simulink model "LKAS_AutoSave_DF_20220408_1006_SW62"  (R2018b)
settings: Solver=FixedStepDiscrete  StartTime=0.0  StopTime=10.0  FixedStep=0.01  RelTol=1e-3
undefined symbols (not defined in the file): LKA_CarWidth, LKA_SampleTime, LKA_StrRatio_C, LKA_Veh2CamL_C, LKA_Veh2CamW_C, LKA_WhlBaseL_C, LL_CompHdAg_C, LL_CompSWA_C, LL_CrvtPrvwT_C, LL_DesDvt_C, LL_DvtComp_C, LL_DvtPrvwT_C, LL_DvtSpdDet_vDvtSpdMin_C, LL_HandsOff_ExitTime, LL_HandsOff_TextTime, LL_HandsOff_WarnTime, LL_HdAgExT_C, LL_HdAgPrvwT_C, LL_LAccMax_C, LL_LAccRMax_C, LL_LDW_EarliestWarnLine_C, LL_LDW_LatestWarnLine_C, LL_LDWS_SUPPRESS_HEADING, LL_LFClb_TFC_FfCtlRatio_C, LL_LFClb_TFC_KdBalance_C, LL_LFClb_TFC_KdMaxSWA_C, LL_LFClb_TFC_KdV1_C, LL_LFClb_TFC_KdV2_C, LL_LFClb_TFC_KdVehSpdLwr_C, LL_LFClb_TFC_KdVehSpdUpr_C, LL_LFClb_TFC_Ki_C, LL_LFClb_TFC_KiMaxSWA_C, LL_LFClb_TFC_Kp_C, LL_LFClb_TFC_KpKlat_C, LL_LFClb_TFC_KpV1_C, LL_LFClb_TFC_KpV2_C, LL_LFClb_TFC_KpVehSpdLwr_C, LL_LFClb_TFC_KpVehSpdUpr_C, LL_LFClb_TFC_PrvwT_C, LL_LKA_EarliestWarnLine_C, LL_LKA_LatestWarnLine_C, LL_LKAExPrcs_ExitC0Dvt, LL_LKAExPrcs_ExitC0Swt, LL_LKAExPrcs_tiExitDelayTime3, LL_LKAExPrcs_tiExitTime1, LL_LKAExPrcs_tiExitTime2, LL_LKAExPrcs_tiExitTime3, LL_LKAS_OUT_OF_CONTROL_LAT_VEL, LL_LKAS_OUT_OF_CONTROL_TTLC, LL_LKASWASyn_M0, LL_LKASWASyn_M1, LL_LKASWASyn_M2, LL_LKASWASyn_M3D, LL_LKASWASyn_M3K_DT, LL_LKASWASyn_M3K_MSD, LL_LKASWASyn_M4K, LL_LKASWASyn_SWAaddMax, LL_LKASWASyn_T2, LL_LKASWASyn_tiTrqSwaRtTime, LL_LKASWASyn_tiTrqSwaTime ... (+47)
libraries: simulink x234, canmsglib x6, dspstat3 x3, simulink_extras x1
(part 7 of 16)

== system LKAS_AutoSave_DF_20220408_1006_SW62/LKAS/LL/LL Inputs Mapping/bsLaneInfo/LanesReconstruct /Right Lane Reconstruct (RgtLaneR) ==
  bsL0Info : Inport
  bsR0Info : Inport  Port=2
  lRoadW : Inport  Port=3
  Add : Sum  OutDataTypeStr=single
  Bus Creator1 : BusCreator  Inputs=8
  Bus Selector1 : BusSelector  OutputSignals=R0_Q
  Bus Selector3 : BusSelector  OutputSignals=L0_C0,L0_C1,L0_C2,L0_C3,L0_VR,L0_Type,L0_W
  Cast To Single{1..4,6} (5 alike) : DataTypeConversion  OutDataTypeStr=single  LockScale=on
  Cast To Single5 : DataTypeConversion  OutDataTypeStr=uint8  LockScale=on
  bsR0InfoR : Outport
  wires:
  Cast To Single4/1 -> Bus Creator1/5  "R0_VR"
  Cast To Single3/1 -> Bus Creator1/4  "R0_C3"
  Cast To Single2/1 -> Bus Creator1/3  "R0_C2"
  Cast To Single1/1 -> Bus Creator1/2  "R0_C1"
  Add/1 -> Bus Creator1/1  "R0_C0"
  Bus Creator1/1 -> bsR0InfoR/1  "bsR0Info"
  Bus Selector1/1 -> Bus Creator1/6  "<R0_Q>"
  bsR0Info/1 -> Bus Selector1/1
  Bus Selector3/5 -> Cast To Single4/1  "<L0_VR>"
  Bus Selector3/4 -> Cast To Single3/1  "<L0_C3>"
  Bus Selector3/3 -> Cast To Single2/1  "<L0_C2>"
  Bus Selector3/2 -> Cast To Single1/1  "<L0_C1>"
  lRoadW/1 -> Add/1
  bsL0Info/1 -> Bus Selector3/1
  Bus Selector3/1 -> Add/2  "<L0_C0>"
  Bus Selector3/6 -> Cast To Single5/1  "<L0_Type>"
  Bus Selector3/7 -> Cast To Single6/1  "<L0_W>"
  Cast To Single5/1 -> Bus Creator1/7  "R0_Type"
  Cast To Single6/1 -> Bus Creator1/8  "R0_W"

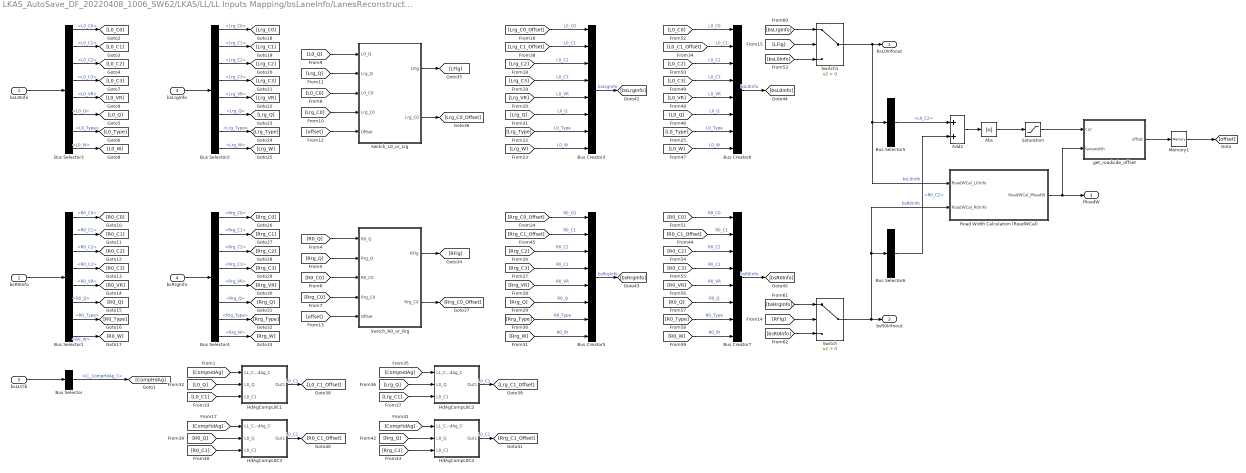
== system LKAS_AutoSave_DF_20220408_1006_SW62/LKAS/LL/LL Inputs Mapping/bsLaneInfo/LanesReconstruct /RoadSide Offset ==
  bsL0Info : Inport
  bsR0Info : Inport  Port=2
  bsLrgInfo : Inport  Port=3
  bsRrgInfo : Inport  Port=4
  bsLLClb : Inport  Port=5
  Abs : Abs
  Add2 : Sum
  Bus Creator{3,5..7} (4 alike) : BusCreator  Inputs=8
  Bus Selector : BusSelector  OutputSignals=bsLKAClb.LL_CompHdAg_C
  Bus Selector1 : BusSelector  OutputSignals=R0_C0,R0_C1,R0_C2,R0_C3,R0_VR,R0_Q,R0_Type,R0_W
  Bus Selector2 : BusSelector  OutputSignals=Lrg_C0,Lrg_C1,Lrg_C2,Lrg_C3,Lrg_VR,Lrg_Q,Lrg_Type,Lrg_W
  Bus Selector3 : BusSelector  OutputSignals=L0_C0,L0_C1,L0_C2,L0_C3,L0_VR,L0_Q,L0_Type,L0_W
  Bus Selector4 : BusSelector  OutputSignals=Rrg_C0,Rrg_C1,Rrg_C2,Rrg_C3,Rrg_VR,Rrg_Q,Rrg_Type,Rrg_W
  Bus Selector5 : BusSelector  OutputSignals=L0_C2
  Bus Selector6 : BusSelector  OutputSignals=R0_C2
  HdAgCompL0C1 : Subsystem
  HdAgCompL0C2 : Subsystem
  HdAgCompL0C3 : Subsystem
  HdAgCompL0C4 : Subsystem
  Memory1 : Memory  InheritSampleTime=on
  Road Width Calculation (RoadWCal) : Subsystem
  Saturation : Saturate  UpperLimit=0.004  LowerLimit=0
      settings: AttributesFormatString="Min = %<LowerLimit>  Max = %<UpperLimit>"
  Switch : Switch  Criteria=u2 > Threshold
  Switch1 : Switch  Criteria=u2 > Threshold
  Switch_L0_or_Lrg : MATLAB Function  TreatAsAtomicUnit=on
  Switch_R0_or_Rrg : MATLAB Function  TreatAsAtomicUnit=on
  get_roadside_offset : MATLAB Function  TreatAsAtomicUnit=on
  bsL0Infoout : Outport
  bsR0Infoout : Outport  Port=2
  lRoadW : Outport  Port=3
  wires:
  Road Width Calculation (RoadWCal)/1(RoadWCal_lRoadW) -> get_roadside_offset/2(lanewidth), lRoadW/1
  Bus Selector6/1 -> Add2/2  "<R0_C2>"
  Bus Selector5/1 -> Add2/1  "<L0_C2>"
  [bsR0Info] -> Switch/3
  Bus Creator7/1 -> [bsR0Info]  "bsR0Info"
  [bsRrgInfo] -> Switch/1
  [bsL0Info] -> Switch1/3
  [bsLrgInfo] -> Switch1/1
  Bus Creator6/1 -> [bsL0Info]  "bsL0Info"
  Bus Creator5/1 -> [bsRrgInfo]  "bsRrgInfo"
  [R0_W] -> Bus Creator7/8  "R0_W"
  [R0_Type] -> Bus Creator7/7  "R0_Type"
  [R0_Q] -> Bus Creator7/6  "R0_Q"
  [R0_VR] -> Bus Creator7/5  "R0_VR"
  [R0_C3] -> Bus Creator7/4  "R0_C3"
  [R0_C2] -> Bus Creator7/3  "R0_C2"
  [R0_C1_Offset] -> Bus Creator7/2  "R0_C1"
  [R0_C0] -> Bus Creator7/1  "R0_C0"
  [L0_W] -> Bus Creator6/8  "L0_W"
  [L0_Type] -> Bus Creator6/7  "L0_Type"
  [L0_Q] -> Bus Creator6/6  "L0_Q"
  [L0_VR] -> Bus Creator6/5  "L0_VR"
  [L0_C3] -> Bus Creator6/4  "L0_C3"
  [L0_C2] -> Bus Creator6/3  "L0_C2"
  [L0_C0] -> Bus Creator6/1  "L0_C0"
  Bus Creator3/1 -> [bsLrgInfo]  "bsLrgInfo"
  [L0_C1_Offset] -> Bus Creator6/2  "L0_C1"
  [CompHdAg] -> HdAgCompL0C3/1(LL_CompHdAg_C)
  [R0_Q] -> HdAgCompL0C3/2(L0_Q)
  [R0_C1] -> HdAgCompL0C3/3(L0_C1)
  HdAgCompL0C3/1(Out1) -> [R0_C1_Offset]  "L0_C1"
  [CompHdAg] -> HdAgCompL0C4/1(LL_CompHdAg_C)
  [Rrg_Q] -> HdAgCompL0C4/2(L0_Q)
  [Rrg_C1] -> HdAgCompL0C4/3(L0_C1)
  HdAgCompL0C4/1(Out1) -> [Rrg_C1_Offset]  "L0_C1"
  HdAgCompL0C2/1(Out1) -> [Lrg_C1_Offset]  "L0_C1"
  [Lrg_C1] -> HdAgCompL0C2/3(L0_C1)
  [Lrg_Q] -> HdAgCompL0C2/2(L0_Q)
  [CompHdAg] -> HdAgCompL0C2/1(LL_CompHdAg_C)
  HdAgCompL0C1/1(Out1) -> [L0_C1_Offset]  "L0_C1"
  [L0_C1] -> HdAgCompL0C1/3(L0_C1)
  [L0_Q] -> HdAgCompL0C1/2(L0_Q)
  [Rrg_C0_Offset] -> Bus Creator5/1  "R0_C0"
  [Rrg_W] -> Bus Creator5/8  "R0_W"
  [Rrg_Type] -> Bus Creator5/7  "R0_Type"
  [Rrg_C1_Offset] -> Bus Creator5/2  "R0_C1"
  [Rrg_C2] -> Bus Creator5/3  "R0_C2"
  [Rrg_C3] -> Bus Creator5/4  "R0_C3"
  [Rrg_VR] -> Bus Creator5/5  "R0_VR"
  [Rrg_Q] -> Bus Creator5/6  "R0_Q"
  [Lrg_Q] -> Bus Creator3/6  "L0_Q"
  [Lrg_VR] -> Bus Creator3/5  "L0_VR"
  [Lrg_C3] -> Bus Creator3/4  "L0_C3"
  [Lrg_C2] -> Bus Creator3/3  "L0_C2"
  [Lrg_C1_Offset] -> Bus Creator3/2  "L0_C1"
  [Lrg_Type] -> Bus Creator3/7  "L0_Type"
  [Lrg_W] -> Bus Creator3/8  "L0_W"
  [Lrg_C0_Offset] -> Bus Creator3/1  "L0_C0"
  Switch_R0_or_Rrg/2(Rrg_C0) -> [Rrg_C0_Offset]
  Switch_L0_or_Lrg/2(Lrg_C0) -> [Lrg_C0_Offset]
  [LFlg] -> Switch1/2
  [RFlg] -> Switch/2
  Switch_L0_or_Lrg/1(LFlg) -> [LFlg]
  Switch_R0_or_Rrg/1(RFlg) -> [RFlg]
  [offset] -> Switch_R0_or_Rrg/5(Offset)
  [offset] -> Switch_L0_or_Lrg/5(Offset)
  [Lrg_Q] -> Switch_L0_or_Lrg/2(Lrg_Q)
  [Lrg_C0] -> Switch_L0_or_Lrg/4("Lrg_C0 ")
  [L0_C0] -> Switch_L0_or_Lrg/3(L0_C0)
  [L0_Q] -> Switch_L0_or_Lrg/1(L0_Q)
  [Rrg_C0] -> Switch_R0_or_Rrg/4("Rrg_C0 ")
  [R0_C0] -> Switch_R0_or_Rrg/3(R0_C0)
  [Rrg_Q] -> Switch_R0_or_Rrg/2(Rrg_Q)
  [R0_Q] -> Switch_R0_or_Rrg/1(R0_Q)
  Bus Selector4/8 -> [Rrg_W]  "<Rrg_W>"
  Bus Selector4/7 -> [Rrg_Type]  "<Rrg_Type>"
  Bus Selector4/6 -> [Rrg_Q]  "<Rrg_Q>"
  Bus Selector4/5 -> [Rrg_VR]  "<Rrg_VR>"
  Bus Selector4/4 -> [Rrg_C3]  "<Rrg_C3>"
  Bus Selector4/3 -> [Rrg_C2]  "<Rrg_C2>"
  Bus Selector4/2 -> [Rrg_C1]  "<Rrg_C1>"
  Bus Selector4/1 -> [Rrg_C0]  "<Rrg_C0>"
  Bus Selector2/8 -> [Lrg_W]  "<Lrg_W>"
  Bus Selector2/7 -> [Lrg_Type]  "<Lrg_Type>"
  Bus Selector2/6 -> [Lrg_Q]  "<Lrg_Q>"
  Bus Selector2/5 -> [Lrg_VR]  "<Lrg_VR>"
  Bus Selector2/4 -> [Lrg_C3]  "<Lrg_C3>"
  Bus Selector2/3 -> [Lrg_C2]  "<Lrg_C2>"
  Bus Selector2/2 -> [Lrg_C1]  "<Lrg_C1>"
  Bus Selector2/1 -> [Lrg_C0]  "<Lrg_C0>"
  Bus Selector1/8 -> [R0_W]  "<R0_W>"
  Bus Selector1/7 -> [R0_Type]  "<R0_Type>"
  Bus Selector1/5 -> [R0_VR]  "<R0_VR>"
  Bus Selector1/6 -> [R0_Q]  "<R0_Q>"
  Bus Selector1/4 -> [R0_C3]  "<R0_C3>"
  Bus Selector1/3 -> [R0_C2]  "<R0_C2>"
  Bus Selector1/2 -> [R0_C1]  "<R0_C1>"
  Bus Selector1/1 -> [R0_C0]  "<R0_C0>"
  Bus Selector3/5 -> [L0_VR]  "<L0_VR>"
  Bus Selector3/8 -> [L0_W]  "<L0_W>"
  Bus Selector3/4 -> [L0_C3]  "<L0_C3>"
  Bus Selector3/7 -> [L0_Type]  "<L0_Type>"
  Bus Selector3/6 -> [L0_Q]  "<L0_Q>"
  Bus Selector3/3 -> [L0_C2]  "<L0_C2>"
  Memory1/1 -> [offset]
  bsRrgInfo/1 -> Bus Selector4/1
  bsLrgInfo/1 -> Bus Selector2/1
  [CompHdAg] -> HdAgCompL0C1/1(LL_CompHdAg_C)
  Bus Selector3/2 -> [L0_C1]  "<L0_C1>"
  Bus Selector/1 -> [CompHdAg]  "<LL_CompHdAg_C>"
  Bus Selector3/1 -> [L0_C0]  "<L0_C0>"
  bsLLClb/1 -> Bus Selector/1
  get_roadside_offset/1(offset) -> Memory1/1
  Saturation/1 -> get_roadside_offset/1(cur)
  Abs/1 -> Saturation/1
  Add2/1 -> Abs/1
  Switch/1 -> bsR0Infoout/1, Bus Selector6/1, Road Width Calculation (RoadWCal)/2(RoadWCal_R0Info)  "bsR0Info"
  bsR0Info/1 -> Bus Selector1/1
  bsL0Info/1 -> Bus Selector3/1
  Switch1/1 -> Bus Selector5/1, Road Width Calculation (RoadWCal)/1(RoadWCal_L0Info), bsL0Infoout/1  "bsL0Info"

== system LKAS_AutoSave_DF_20220408_1006_SW62/LKAS/LL/LLOn/LDW/Heading Angle Detection (HdAgDet)/If Action Subsystem ==
  In1 : Inport
  Action Port : ActionPort  InitializeStates=reset  ActionType=then
      settings: AttributesFormatString=states = %<InitializeStates>
  Gain : Gain  Gain=-1  OutDataTypeStr=single
  rad to deg : Gain  Gain=180/pi  OutDataTypeStr=single
  Out1 : Outport  InitialOutput=0
      settings: AttributesFormatString=%<OutputWhenDisabled> = %<InitialOutput>
  wires:
  rad to deg/1 -> Out1/1
  Gain/1 -> rad to deg/1
  In1/1 -> Gain/1

== system LKAS_AutoSave_DF_20220408_1006_SW62/LKAS/LL/LLOn/LDW/Heading Angle Detection (HdAgDet)/If Action Subsystem1 ==
  In1 : Inport
  Action Port : ActionPort  InitializeStates=reset  ActionType=elseif
      settings: AttributesFormatString=states = %<InitializeStates>
  rad to deg : Gain  Gain=180/pi  OutDataTypeStr=single
  Out1 : Outport  InitialOutput=0
      settings: AttributesFormatString=%<OutputWhenDisabled> = %<InitialOutput>
  wires:
  rad to deg/1 -> Out1/1
  In1/1 -> rad to deg/1

== system LKAS_AutoSave_DF_20220408_1006_SW62/LKAS/LL/LLOn/LDW/Heading Angle Detection (HdAgDet)/If Action Subsystem2 ==
  Action Port : ActionPort  InitializeStates=reset  ActionType=else
      settings: AttributesFormatString=states = %<InitializeStates>
  Constant : Constant  Value=0  OutDataTypeStr=single
  Out1 : Outport  InitialOutput=0
      settings: AttributesFormatString=%<OutputWhenDisabled> = %<InitialOutput>
  wires:
  Constant/1 -> Out1/1

== system LKAS_AutoSave_DF_20220408_1006_SW62/LKAS/LL/LLOn/LDW/Heading Angle Detection (HdAgDet)/Sum Condition ==
  In : Inport
  Sum : Inport  Port=2
  Enable : EnablePort  StatesWhenEnabling=reset
      settings: AttributesFormatString=states = %<StatesWhenEnabling>
  Add1 : Sum  OutDataTypeStr=single
  Memory : Memory  InheritSampleTime=on
  Relational Operator : RelationalOperator  OutDataTypeStr=boolean  RndMeth=Nearest
  Saturation : Saturate  UpperLimit=0.6  LowerLimit=0
      settings: AttributesFormatString="Min = %<LowerLimit>  Max = %<UpperLimit>"
  Out : Outport  OutputWhenDisabled=reset  InitialOutput=0
      settings: AttributesFormatString=%<OutputWhenDisabled> = %<InitialOutput>
  wires:
  Saturation/1 -> Relational Operator/1, Memory/1
  Sum/1 -> Relational Operator/2
  In/1 -> Add1/1
  Add1/1 -> Saturation/1
  Memory/1 -> Add1/2
  Relational Operator/1 -> Out/1

== system LKAS_AutoSave_DF_20220408_1006_SW62/LKAS/LL/LLOn/LKA/Driver Torque Addition (DTA)/Driver Torque Assist ==
  DTA_bsInInfoSyn : Inport
  DTA_bsLFClb : Inport  Port=2
  DTA_Exit3Flg : Inport  Port=3
  Abs : Abs
  Add : Sum  Inputs=+-
  Add1 : Sum  Inputs=--+
  Bus Selector : BusSelector  OutputSignals=bsEPSInfo.EPS_SW_Trq
  Bus Selector1 : BusSelector  OutputSignals=bsLKAClb.LL_LKASWAClb.LL_LKASWASyn_M3D,bsLKAClb.LL_LKASWAClb.LL_LKASWASyn_M3K_DT,bsLKAClb.LL_LKASWAClb.LL_LKASWASyn_M3K_MSD,bsLKAClb.LL_LKASWAClb.LL_LKASWASyn_M0,bsLKAClb.LL_LKASWAClb.LL_LKASWASyn_M1,bsLKAClb.LL_LKASWAClb.LL_LKASWASyn_M2,bsLKAClb.LL_LKASWAClb.LL_LKASWASyn_T2,bsLKAClb.LL_LKASWAClb.LL_LKASWASyn_M4K,bsLKAClb.LL_LKAExPrcs.LL_LKAExPrcs_tiExitDelayTime3
  Divide : Product  Inputs=**
  Divide1 : Product  Inputs=**
  Divide2 : Product  Inputs=*/
  Divide5 : Product  Inputs=**
  MATLAB Function : MATLAB Function  TreatAsAtomicUnit=on
  Moving Standard Deviation2 : Subsystem  TreatAsAtomicUnit=on
      mask Display: disp(['Moving' char(10) 'Standard' char(10) 'Deviation']);
  Saturation1 : Saturate  UpperLimit=0.4  LowerLimit=0
      settings: AttributesFormatString="Min = %<LowerLimit>  Max = %<UpperLimit>"
  Saturation2 : Saturate  UpperLimit=1  LowerLimit=0.01
      settings: AttributesFormatString="Min = %<LowerLimit>  Max = %<UpperLimit>"
  Saturation3 : Saturate  UpperLimit=0.4  LowerLimit=0
      settings: AttributesFormatString="Min = %<LowerLimit>  Max = %<UpperLimit>"
  Saturation4 : Saturate  UpperLimit=2  LowerLimit=0
      settings: AttributesFormatString="Min = %<LowerLimit>  Max = %<UpperLimit>"
  Saturation5 : Saturate  UpperLimit=1  LowerLimit=0
      settings: AttributesFormatString="Min = %<LowerLimit>  Max = %<UpperLimit>"
  Saturation6 : Saturate  UpperLimit=1  LowerLimit=0.01
      settings: AttributesFormatString="Min = %<LowerLimit>  Max = %<UpperLimit>"
  Saturation7 : Saturate  UpperLimit=1  LowerLimit=0
      settings: AttributesFormatString="Min = %<LowerLimit>  Max = %<UpperLimit>"
  Sum Condition2 : Subsystem  TreatAsAtomicUnit=on
  TickTime (TTime) : Subsystem
      mask Display:
      | port_label('output', 1, 'TTime');
      | color('blue');
      | text(0.98,0.9,'VCDC Block','horizontalAlignment','right');
      | color('black');
      | text(0.5,0.55,'Tick Time','horizontalAlignment','center');
      | text(0.5,0.4,'(TTime)','horizontalAlignment','center');
  DTA_M : Outport
      settings: AttributesFormatString=%<OutputWhenDisabled> = %<InitialOutput>
  wires:
  Abs/1 -> Saturation7/1
  Saturation4/1 -> Abs/1
  Add1/1 -> Saturation6/1
  Divide5/1 -> Saturation2/1
  Sum Condition2/1(M4K) -> Divide5/2
  Bus Selector1/9 -> Sum Condition2/3(Sum)  "<LL_LKAExPrcs_tiExitDelayTime3>"
  [LKA_SampleTime] -> Sum Condition2/1(SampleTime)
  DTA_Exit3Flg/1 -> Sum Condition2/Enable
  Bus Selector1/8 -> Sum Condition2/2(LL_LKASWASyn_M4K)  "<LL_LKASWASyn_M4K>"
  Bus Selector1/3 -> Divide/2  "<LL_LKASWASyn_M3K_MSD>"
  Bus Selector1/2 -> Divide1/2  "<LL_LKASWASyn_M3K_DT>"
  Moving Standard Deviation2/1(Out2) -> Add/2  "DT"
  Saturation2/1 -> DTA_M/1
  DTA_bsLFClb/1 -> Bus Selector1/1
  DTA_bsInInfoSyn/1 -> Bus Selector/1
  Moving Standard Deviation2/2(Out1) -> Divide/1  "MSD"
  Bus Selector/1 -> Add/1, Moving Standard Deviation2/1(In1)  "<EPS_SW_Trq>"
  Bus Selector1/6 -> MATLAB Function/3(M2)  "<LL_LKASWASyn_M2>"
  Saturation6/1 -> Divide5/1
  Divide/1 -> Saturation1/1
  TickTime (TTime)/1(Out1) -> [T]
  Bus Selector1/7 -> ?  "<LL_LKASWASyn_T2>"
  MATLAB Function/1(M) -> Add1/3
  Saturation1/1 -> Add1/2  "M3_MSD"
  [T] -> MATLAB Function/6(T)
  [PT1] -> MATLAB Function/4(T1), MATLAB Function/5(T2)
  Bus Selector1/5 -> MATLAB Function/2(M1)  "<LL_LKASWASyn_M1>"
  Bus Selector1/4 -> MATLAB Function/1(M0)  "<LL_LKASWASyn_M0>"
  Add/1 -> Saturation4/1
  Divide1/1 -> Saturation3/1
  Saturation7/1 -> Divide2/1
  Divide2/1 -> Saturation5/1
  Bus Selector1/1 -> Divide2/2  "<LL_LKASWASyn_M3D>"
  Saturation3/1 -> Add1/1  "M3_DT"
  Saturation5/1 -> Divide1/1

== system LKAS_AutoSave_DF_20220408_1006_SW62/LKAS/LL/LLOn/LKA/Driver Torque Addition (DTA)/Subsystem ==
  DTA_bsInInfoSyn : Inport
  DTA_bsLFClb : Inport  Port=2
  Enable : EnablePort
      settings: AttributesFormatString=states = %<StatesWhenEnabling>
  Add : Sum
  Bus Selector2 : BusSelector  OutputSignals=bsVehMovInfo.ESC_VehSpd,bsEPSInfo.EPS_SW_Trq,bsLaneInfo.bsL0Info.L0_C0,bsLaneInfo.bsR0Info.R0_C0
  Bus Selector4 : BusSelector  OutputSignals=bsLKAClb.LL_LKASWAClb.LL_LKASWASyn_SWAaddMax,bsLKAClb.LL_LKASWAClb.LL_LKASWASyn_TrqMax,bsLKAClb.LL_LKASWAClb.LL_LKASWASyn_TrqSwaAddSwt,bsLKAClb.LL_LKASWAClb.LL_LKASWASyn_tiTrqSwaTime,bsLKAClb.LL_LKASWAClb.LL_LKASWASyn_tiTrqSwaRtTime,bsLKAClb.LL_LKASWAClb.LL_LKASWASyn_TrqSwaRateDiff,bsConstantClb.LKA_SampleTime
  Constant1 : Constant  Value=5  OutDataTypeStr=single
  Constant2 : Constant  Value=-5  OutDataTypeStr=single
  Divide1 : Product  Inputs=***
  Divide3 : Product  Inputs=**
  DriverSwaTrqAdd : MATLAB Function  TreatAsAtomicUnit=on
  LowPass : Subsystem
  LowPass1 : Subsystem
  Rate Limiter Dynamic : simulink/Discontinuities/Rate Limiter Dynamic
      settings: SourceProductName=Simulink
  Saturation : Saturate  UpperLimit=30  LowerLimit=-30
      settings: AttributesFormatString="Min = %<LowerLimit>  Max = %<UpperLimit>"
  DTA_phiDTASWACmd : Outport  OutputWhenDisabled=reset  InitialOutput=0
      settings: AttributesFormatString=%<OutputWhenDisabled> = %<InitialOutput>
  wires:
  DTA_bsLFClb/1 -> Bus Selector4/1
  Bus Selector4/2 -> DriverSwaTrqAdd/6(trqmax)  "<LL_LKASWASyn_TrqMax>"
  Bus Selector4/7 -> LowPass/3(dT), LowPass1/3(dT)  "<LKA_SampleTime>"
  Bus Selector2/3 -> DriverSwaTrqAdd/3(l0c0)  "<L0_C0>"
  Bus Selector4/5 -> LowPass1/1(T)  "<LL_LKASWASyn_tiTrqSwaRtTime>"
  Bus Selector2/1 -> DriverSwaTrqAdd/1(spd)  "<ESC_VehSpd>"
  Bus Selector4/6 -> Divide1/3  "<LL_LKASWASyn_TrqSwaRateDiff>"
  Bus Selector2/4 -> DriverSwaTrqAdd/4(r0c0)  "<R0_C0>"
  Bus Selector2/2 -> DriverSwaTrqAdd/2(trq)  "<EPS_SW_Trq>"
  Divide1/1 -> Add/2  "SWARateAdd"
  LowPass/1(y) -> LowPass1/2(u), Divide3/2  "TrqSWAAdd"
  Bus Selector4/4 -> LowPass/1(T)  "<LL_LKASWASyn_tiTrqSwaTime>"
  DTA_bsInInfoSyn/1 -> Bus Selector2/1
  Saturation/1 -> Divide1/2
  Rate Limiter Dynamic/1 -> DTA_phiDTASWACmd/1
  DriverSwaTrqAdd/1(Swaadd) -> LowPass/2(u)  "TrqSWAAddRaw"
  Constant1/1 -> Rate Limiter Dynamic/1
  Bus Selector4/1 -> DriverSwaTrqAdd/5(swaaddmax)  "<LL_LKASWASyn_SWAaddMax>"
  Constant2/1 -> Rate Limiter Dynamic/3
  Divide3/1 -> Add/1  "TrqSWAAdd"
  LowPass1/1(y) -> Saturation/1  "SWARateAdd"
  Bus Selector4/3 -> Divide1/1, Divide3/1  "<LL_LKASWASyn_TrqSwaAddSwt>"
  Add/1 -> Rate Limiter Dynamic/2

== system LKAS_AutoSave_DF_20220408_1006_SW62/LKAS/LL/LLOn/LKA/LKA Exit Processing (LKAExPrcs)/Exit Time 1 ==
  bsLKAInPInfo : Inport
  bsLKAClb : Inport  Port=2
  Abs : Abs
  Add : Sum
  Add2 : Sum  OutDataTypeStr=single
  Bus Selector1 : BusSelector  OutputSignals=bsConstantClb.LKA_SampleTime,bsLKAClb.LL_LKAExPrcs.LL_LKAExPrcs_tiExitTime1
  Bus Selector2 : BusSelector  OutputSignals=bsPrCrvtInfo.crPrvwCrvt
  Constant : Constant  Value=0.004  OutDataTypeStr=single
  Constant1 : Constant  Value=0.5  OutDataTypeStr=single
  Divide : Product  Inputs=***/
  Memory : Memory  InheritSampleTime=on
  Relational Operator4 : RelationalOperator  OutDataTypeStr=boolean  RndMeth=Nearest
  Saturation : Saturate  UpperLimit=0.004  LowerLimit=0
      settings: AttributesFormatString="Min = %<LowerLimit>  Max = %<UpperLimit>"
  Saturation2 : Saturate  UpperLimit=20  LowerLimit=0
      settings: AttributesFormatString="Min = %<LowerLimit>  Max = %<UpperLimit>"
  Exit1 : Outport
  wires:
  Bus Selector1/2 -> Divide/1, Add/1  "<LL_LKAExPrcs_tiExitTime1>"
  Saturation/1 -> Divide/3
  Add/1 -> Relational Operator4/2
  Abs/1 -> Saturation/1
  Divide/1 -> Add/2
  Bus Selector2/1 -> Abs/1  "<crPrvwCrvt>"
  Constant1/1 -> Divide/2
  Constant/1 -> Divide/4
  bsLKAInPInfo/1 -> Bus Selector2/1
  Relational Operator4/1 -> Exit1/1
  Memory/1 -> Add2/2
  Add2/1 -> Saturation2/1
  bsLKAClb/1 -> Bus Selector1/1
  Bus Selector1/1 -> Add2/1  "<LKA_SampleTime>"
  Saturation2/1 -> Memory/1, Relational Operator4/1

== system LKAS_AutoSave_DF_20220408_1006_SW62/LKAS/LL/LLOn/LKA/LKA Exit Processing (LKAExPrcs)/Exit Time 2 ==
  bsLKAClb : Inport
  bsLKAInPInfo : Inport  Port=2
  T1 : Inport  Port=3
  Abs : Abs
  Abs2 : Abs
  Abs3 : Abs
  Add1 : Sum
  Add2 : Sum  OutDataTypeStr=single
  Add3 : Sum  Inputs=+-
  Bus Selector1 : BusSelector  OutputSignals=bsPrCrvtInfo.crPrvwCrvt
  Bus Selector3 : BusSelector  OutputSignals=bsConstantClb.LKA_SampleTime,bsConstantClb.LKA_CarWidth,bsLKAClb.LL_LKAExPrcs.LL_LKAExPrcs_tiExitTime2
  Bus Selector4 : BusSelector  OutputSignals=bsDvtInfo.ILftDvt,bsDvtInfo.IRgtDvt,LaneWidth
  Constant : Constant  Value=0.004  OutDataTypeStr=single
  Constant1 : Constant  Value=0.5  OutDataTypeStr=single
  Divide : Product  Inputs=***/
  Gain : Gain  Gain=1/6
  Logical Operator1 : Logic  Inputs=3  AllPortsSameDT=off  OutDataTypeStr=boolean
  Memory : Memory  InheritSampleTime=on
  Relational Operator2 : RelationalOperator  OutDataTypeStr=boolean  RndMeth=Nearest
  Relational Operator3 : RelationalOperator  OutDataTypeStr=boolean  RndMeth=Nearest
  Relational Operator4 : RelationalOperator  OutDataTypeStr=boolean  RndMeth=Nearest
  Saturation : Saturate  UpperLimit=0.004  LowerLimit=0
      settings: AttributesFormatString="Min = %<LowerLimit>  Max = %<UpperLimit>"
  Saturation2 : Saturate  UpperLimit=12  LowerLimit=0
      settings: AttributesFormatString="Min = %<LowerLimit>  Max = %<UpperLimit>"
  Sum Condition1 : Subsystem
  Exit2 : Outport
  wires:
  Bus Selector3/3 -> Divide/1, Add1/1  "<LL_LKAExPrcs_tiExitTime2>"
  Bus Selector3/2 -> Add3/2  "<LKA_CarWidth>"
  bsLKAClb/1 -> Bus Selector3/1
  Saturation/1 -> Divide/3
  Divide/1 -> Add1/2
  Constant1/1 -> Divide/2
  Abs/1 -> Saturation/1
  Constant/1 -> Divide/4
  Add1/1 -> Sum Condition1/2(Time Exit 2)
  Bus Selector1/1 -> Abs/1  "<crPrvwCrvt>"
  bsLKAInPInfo/1 -> Bus Selector4/1, Bus Selector1/1
  Sum Condition1/1(Out) -> Exit2/1
  T1/1 -> Relational Operator4/2
  Bus Selector3/1 -> Add2/1, Sum Condition1/1(Sample Time)  "<LKA_SampleTime>"
  Memory/1 -> Add2/2
  Relational Operator4/1 -> Logical Operator1/1
  Add2/1 -> Saturation2/1
  Logical Operator1/1 -> Sum Condition1/Enable
  Relational Operator3/1 -> Logical Operator1/3
  Abs2/1 -> Relational Operator2/1
  Relational Operator2/1 -> Logical Operator1/2
  Abs3/1 -> Relational Operator3/1
  Gain/1 -> Relational Operator3/2, Relational Operator2/2
  Saturation2/1 -> Memory/1, Relational Operator4/1
  Bus Selector4/1 -> Abs2/1  "<ILftDvt>"
  Bus Selector4/2 -> Abs3/1  "<IRgtDvt>"
  Bus Selector4/3 -> Add3/1  "<LaneWidth>"
  Add3/1 -> Gain/1

== system LKAS_AutoSave_DF_20220408_1006_SW62/LKAS/LL/LLOn/LKA/LKA Exit Processing (LKAExPrcs)/Exit Time 3 ==
  bsLKAInPInfo : Inport
  bsLKAClb : Inport  Port=2
  T1 : Inport  Port=3
  Abs4 : Abs
  Add : Sum  Inputs=+-
  Add2 : Sum  OutDataTypeStr=single
  Add6 : Sum
  Bus Selector3 : BusSelector  OutputSignals=bsConstantClb.LKA_SampleTime,bsConstantClb.LKA_CarWidth,bsLKAClb.LL_LKAExPrcs.LL_LKAExPrcs_tiExitTime3,bsLKAClb.LL_LKAExPrcs.LL_LKAExPrcs_ExitC0Dvt,bsLKAClb.LL_LKAExPrcs.LL_LKAExPrcs_ExitC0Swt,bsLKAClb.LL_LKAExPrcs.LL_LKAExPrcs_tiExitDelayTime3
  Bus Selector4 : BusSelector  OutputSignals=bsPrCrvtInfo.crPrvwCrvt
  Bus Selector5 : BusSelector  OutputSignals=LaneWidth,bsDvtInfo.ILftDvt,bsDvtInfo.IRgtDvt
  Constant : Constant  Value=0.004  OutDataTypeStr=single
  Constant7 : Constant  Value=2  OutDataTypeStr=single
  Detect Rise Positive : simulink/Logic and Bit Operations/Detect Rise Positive  vinit=0  OutDataTypeStr=boolean
  Divide1 : Product  Inputs=**/
  Gain : Gain  Gain=1/3
  If : If  IfExpression=u1
  If Action Subsystem : Subsystem  TreatAsAtomicUnit=on
  If Action Subsystem3 : Subsystem  TreatAsAtomicUnit=on
  Logical Operator1 : Logic  Inputs=3  AllPortsSameDT=off  OutDataTypeStr=boolean
  Logical Operator2 : Logic  Inputs=4  AllPortsSameDT=off  OutDataTypeStr=boolean
  Memory : Memory  InheritSampleTime=on
  Memory1 : Memory  InheritSampleTime=on
  Merge : Merge
  Moving Standard Deviation1 : Subsystem  TreatAsAtomicUnit=on
      mask Display: disp(['Moving' char(10) 'Standard' char(10) 'Deviation']);
  Moving Standard Deviation2 : Subsystem  TreatAsAtomicUnit=on
      mask Display: disp(['Moving' char(10) 'Standard' char(10) 'Deviation']);
  Relational Operator2 : RelationalOperator  OutDataTypeStr=boolean  RndMeth=Nearest
  Relational Operator3 : RelationalOperator  OutDataTypeStr=boolean  RndMeth=Nearest
  Relational Operator4 : RelationalOperator  OutDataTypeStr=boolean  RndMeth=Nearest
  Relational Operator5 : RelationalOperator  Operator=<=  OutDataTypeStr=boolean  RndMeth=Nearest
  Relational Operator6 : RelationalOperator  Operator=<=  OutDataTypeStr=boolean  RndMeth=Nearest
  Saturation : Saturate  UpperLimit=0.004  LowerLimit=0
      settings: AttributesFormatString="Min = %<LowerLimit>  Max = %<UpperLimit>"
  Saturation2 : Saturate  UpperLimit=10  LowerLimit=0
      settings: AttributesFormatString="Min = %<LowerLimit>  Max = %<UpperLimit>"
  Sum Condition : Subsystem
  Sum Condition1 : Subsystem
  Sum Condition2 : Subsystem  TreatAsAtomicUnit=on
  Exit3 : Outport
  Exit3_flg : Outport  Port=2
  wires:
  Bus Selector3/6 -> Sum Condition2/2(Sum)  "<LL_LKAExPrcs_tiExitDelayTime3>"
  Detect Rise Positive/1 -> If/1
  If Action Subsystem/1(Out) -> Merge/1
  [LKA_SampleTime] -> Sum Condition2/1(SampleTime)
  Memory1/1 -> If Action Subsystem3/1(In1)
  Logical Operator2/1 -> Detect Rise Positive/1
  Sum Condition2/1(Out) -> Exit3/1
  Merge/1 -> Memory1/1, Sum Condition2/Enable, Exit3_flg/1
  If/2 -> If Action Subsystem3/Action
  If Action Subsystem3/1(Out) -> Merge/2
  If/1 -> If Action Subsystem/Action
  Bus Selector3/1 -> [LKA_SampleTime]  "<LKA_SampleTime>"
  Bus Selector3/2 -> Add/2  "<LKA_CarWidth>"
  Bus Selector3/3 -> Add6/1  "<LL_LKAExPrcs_tiExitTime3>"
  Bus Selector3/4 -> Relational Operator5/2, Relational Operator6/2  "<LL_LKAExPrcs_ExitC0Dvt>"
  Bus Selector3/5 -> Logical Operator2/4  "<LL_LKAExPrcs_ExitC0Swt>"
  [LKA_SampleTime] -> Sum Condition/1(In), Sum Condition1/1(In)
  Constant7/1 -> Divide1/1
  Bus Selector4/1 -> Abs4/1  "<crPrvwCrvt>"
  Saturation/1 -> Divide1/2
  Abs4/1 -> Saturation/1
  Divide1/1 -> Add6/2
  Constant/1 -> Divide1/3
  bsLKAInPInfo/1 -> Bus Selector5/1, Bus Selector4/1
  Moving Standard Deviation1/1(Out1) -> Relational Operator6/1
  Add6/1 -> Sum Condition1/2(In1), Sum Condition/2(In1)
  Relational Operator6/1 -> Sum Condition1/Enable
  Sum Condition1/1(Out) -> Logical Operator2/2
  Sum Condition/1(Out) -> Logical Operator2/3
  Relational Operator5/1 -> Sum Condition/Enable
  Moving Standard Deviation2/1(Out1) -> Relational Operator5/1
  bsLKAClb/1 -> Bus Selector3/1
  Add/1 -> Gain/1
  Relational Operator2/1 -> Logical Operator1/2
  Relational Operator3/1 -> Logical Operator1/3
  Logical Operator1/1 -> Logical Operator2/1
  Saturation2/1 -> Memory/1, Relational Operator4/1
  Relational Operator4/1 -> Logical Operator1/1
  Add2/1 -> Saturation2/1
  Memory/1 -> Add2/2
  [LKA_SampleTime] -> Add2/1
  T1/1 -> Relational Operator4/2
  Bus Selector5/3 -> Relational Operator3/1, Moving Standard Deviation1/1(In1)  "<IRgtDvt>"
  Bus Selector5/2 -> Relational Operator2/1, Moving Standard Deviation2/1(In1)  "<ILftDvt>"
  Bus Selector5/1 -> Add/1  "<LaneWidth>"
  Gain/1 -> Relational Operator3/2, Relational Operator2/2

== system LKAS_AutoSave_DF_20220408_1006_SW62/LKAS/LL/LLOn/LKA/LKA Motion Planning (LKAMP) /LKA Motion Planning Calculation (LKAMPCal) ==
  LKAMPCal_bsLKAInPInfo : Inport
  LKAMPCal_bsLKAClb : Inport  Port=2
  Action Port : ActionPort  InitializeStates=reset  ActionType=then
      settings: AttributesFormatString=states = %<InitializeStates>
  Bus Creator : BusCreator  Inputs=3
  Bus Selector : BusSelector  OutputSignals=MPInP_stLDDir,MPInP_tiTTLCIni,MPInP_vVehSpdIni,MPInP_phiSWAIni,MPInP_phiPrvwHdAgIni,MPInP_dphiSWARMax,MPInP_StbFacm_SY
  Bus Selector1 : BusSelector  OutputSignals=bsConstantClb.LKA_WhlBaseL_C,bsConstantClb.LKA_StrRatio_C
  MATLAB Function : MATLAB Function  Commented=on  TreatAsAtomicUnit=on
  MATLABFunction1 : MATLAB Function  TreatAsAtomicUnit=on
  LKAMPCal_bsLKAMPCalOut : Outport
      settings: AttributesFormatString=%<OutputWhenDisabled> = %<InitialOutput>
  wires:
  MATLABFunction1/3(K1K2Det_T1) -> Bus Creator/3
  Bus Selector1/2 -> MATLABFunction1/9(K1K2Det_bsSysCfg_SY_StRatio_SY)  "<LKA_StrRatio_C>"
  Bus Selector1/1 -> MATLABFunction1/8(K1K2Det_bsSysCfg_SY_WhlBase_SY)  "<LKA_WhlBaseL_C>"
  LKAMPCal_bsLKAInPInfo/1 -> Bus Selector/1
  LKAMPCal_bsLKAClb/1 -> Bus Selector1/1
  Bus Creator/1 -> LKAMPCal_bsLKAMPCalOut/1  "LKAMPCal_bsLKAMPCalOut"
  MATLABFunction1/1(K1K2Det_dphi1PhSWAGrad) -> Bus Creator/1
  Bus Selector/3 -> MATLABFunction1/3(K1K2Det_vVehSpd)  "<MPInP_vVehSpdIni>"
  Bus Selector/1 -> MATLABFunction1/1(K1K2Det_stLDDir)  "<MPInP_stLDDir>"
  Bus Selector/7 -> MATLABFunction1/7(K1K2Det_bsSysCfg_SY_StbFacm_SY)  "<MPInP_StbFacm_SY>"
  Bus Selector/4 -> MATLABFunction1/4(K1K2Det_phiIniSWA)  "<MPInP_phiSWAIni>"
  MATLABFunction1/2(K1K2Det_phi2PhSWAIni) -> Bus Creator/2
  Bus Selector/2 -> MATLABFunction1/2(K1K2Det_tiTTLC0)  "<MPInP_tiTTLCIni>"
  Bus Selector/5 -> MATLABFunction1/5(K1K2Det_phiPrvwHdAgIni)  "<MPInP_phiPrvwHdAgIni>"
  Bus Selector/6 -> MATLABFunction1/6(K1K2Det_dphiSWARMax)  "<MPInP_dphiSWARMax>"

== system LKAS_AutoSave_DF_20220408_1006_SW62/LKAS/LL/LLOn/LKA/LKA Motion Planning (LKAMP) /Motion Planning Input Processing (MPInP) ==
  MPInP_Ff : Inport
  MPInP_stLKAActvFlg : Inport  Port=2
  MPInP_phiHdAgMax : Inport  Port=3
  MPInP_bsLKAInPInfo : Inport  Port=4
  MPInP_bsInInfoSyn : Inport  Port=5
  Add : Sum  Inputs=+-
  Add1 : Sum  Inputs=+--
  Bus Creator : BusCreator  Inputs=11
  Bus Selector1 : BusSelector  OutputSignals=bsTTLCInfo.LFTTTLC,bsTTLCInfo.RGTTTLC
  Bus Selector3 : BusSelector  OutputSignals=bsSWAInfo.SW_Angle,bsVehMovInfo.ESC_VehSpd
  Bus Selector4 : BusSelector  OutputSignals=bsPrHdAgInfo.lPrvwZLft,bsPrHdAgInfo.lPrvwZRgt,bsPrCrvtInfo.crPrvwCrvtMean,bsUndrLimInfo.UndrLim_dphiSWARMax,bsPrHdAgInfo.phiPrvwTTLCHdAgLftTTLCLft,bsPrHdAgInfo.phiPrvwTTLCHdAgLftTTLCRgt,bsPrHdAgInfo.phiPrvwTTLCHdAgRgtTTLCLft,bsPrHdAgInfo.phiPrvwTTLCHdAgRgtTTLCRgt,bsPrDvtInfo.lPrvwDvtLft,bsPrDvtInfo.lPrvwDvtRgt,bsHdAgInfo.phiHdAg_Lft,bsHdAgInfo.phiHdAg_Rgt,phiSWAPos
  Cast To Single1 : DataTypeConversion  LockScale=on
  Constant : Constant  Value=0.09  OutDataTypeStr=single
  Divide1 : Product  Inputs=*/
  Divide2 : Product  Inputs=**
  Gain : Gain
  Lane Information Selection (LaneInfoSel) : Subsystem
  Lane Information Selection (LaneInfoSel)1 : Subsystem
  Lane Information Selection (LaneInfoSel)2 : Subsystem
  Lane Information Selection (LaneInfoSel)3 : Subsystem
  Lane Information Selection (LaneInfoSel)4 : Subsystem
  Saturation1 : Saturate  UpperLimit=0.0117  LowerLimit=0.00237
      settings: AttributesFormatString="Min = %<LowerLimit>  Max = %<UpperLimit>"
  Saturation2 : Saturate  UpperLimit=2  LowerLimit=0.6
      settings: AttributesFormatString="Min = %<LowerLimit>  Max = %<UpperLimit>"
  Saturation3 : Saturate  UpperLimit=150  LowerLimit=60
      settings: AttributesFormatString="Min = %<LowerLimit>  Max = %<UpperLimit>"
  Signal Latching : Subsystem  mask(Signal Latching:){LatchTime=1}
      mask prompts: LatchTime "Latch time(-):"
      mask help:
      | If the latch time is not reached, the input signal will just go through the block. If the latch time is reached, the output will be held and do not change again. The latch time is described with the number of the sampling time.
      | ----vcdc.ascl@jlu 19-01-15
  Signal Latching2 : Subsystem  mask(Signal Latching:){LatchTime=1}
      mask prompts: LatchTime "Latch time(-):"
      mask help:
      | If the latch time is not reached, the input signal will just go through the block. If the latch time is reached, the output will be held and do not change again. The latch time is described with the number of the sampling time.
      | ----vcdc.ascl@jlu 19-01-15
  Signal Latching3 : Subsystem  mask(Signal Latching:){LatchTime=1}
      mask prompts: LatchTime "Latch time(-):"
      mask help:
      | If the latch time is not reached, the input signal will just go through the block. If the latch time is reached, the output will be held and do not change again. The latch time is described with the number of the sampling time.
      | ----vcdc.ascl@jlu 19-01-15
  Signal Latching4 : Subsystem  mask(Signal Latching:){LatchTime=1}
      mask prompts: LatchTime "Latch time(-):"
      mask help:
      | If the latch time is not reached, the input signal will just go through the block. If the latch time is reached, the output will be held and do not change again. The latch time is described with the number of the sampling time.
      | ----vcdc.ascl@jlu 19-01-15
  Signal Latching5 : Subsystem  mask(Signal Latching:){LatchTime=1}
      mask prompts: LatchTime "Latch time(-):"
      mask help:
      | If the latch time is not reached, the input signal will just go through the block. If the latch time is reached, the output will be held and do not change again. The latch time is described with the number of the sampling time.
      | ----vcdc.ascl@jlu 19-01-15
  Signal Latching6 : Subsystem  mask(Signal Latching:){LatchTime=1}
      mask prompts: LatchTime "Latch time(-):"
      mask help:
      | If the latch time is not reached, the input signal will just go through the block. If the latch time is reached, the output will be held and do not change again. The latch time is described with the number of the sampling time.
      | ----vcdc.ascl@jlu 19-01-15
  Signal Latching7 : Subsystem  mask(Signal Latching:){LatchTime=1}
      mask prompts: LatchTime "Latch time(-):"
      mask help:
      | If the latch time is not reached, the input signal will just go through the block. If the latch time is reached, the output will be held and do not change again. The latch time is described with the number of the sampling time.
      | ----vcdc.ascl@jlu 19-01-15
  Subsystem : Subsystem
  MPInP_bsMPInPInfo : Outport
  wires:
  Bus Selector4/13 -> Add1/3  "<phiSWAPos>"
  Gain/1 -> Bus Creator/6  "MPInP_dphiSWARMax"
  Bus Selector4/7 -> Lane Information Selection (LaneInfoSel)1/4(LaneInfoSel_phiPrvwTTLCHdAgRgtTTLCLft)  "<phiPrvwTTLCHdAgRgtTTLCLft>"
  Bus Selector4/6 -> Lane Information Selection (LaneInfoSel)1/3(LaneInfoSel_phiPrvwTTLCHdAgLftTTLCRgt)  "<phiPrvwTTLCHdAgLftTTLCRgt>"
  Bus Selector4/1 -> Lane Information Selection (LaneInfoSel)3/2(LaneInfoSel_facmLftLane)  "<lPrvwZLft>"
  Lane Information Selection (LaneInfoSel)4/1(LaneInfoSel_facmActvLane) -> Signal Latching4/1(In)  "MPInP_phiHdAgIni"
  Bus Selector4/12 -> Lane Information Selection (LaneInfoSel)4/3(LaneInfoSel_facmRgtLane)  "<phiHdAg_Rgt>"
  Bus Selector4/11 -> Lane Information Selection (LaneInfoSel)4/2(LaneInfoSel_facmLftLane)  "<phiHdAg_Lft>"
  Bus Selector4/2 -> Lane Information Selection (LaneInfoSel)3/3(LaneInfoSel_facmRgtLane)  "<lPrvwZRgt>"
  Add1/1 -> Signal Latching6/1(In)
  MPInP_Ff/1 -> Add1/2
  Add/1 -> Signal Latching2/1(In)
  Bus Selector4/3 -> Divide2/1  "<crPrvwCrvtMean>"
  Lane Information Selection (LaneInfoSel)3/1(LaneInfoSel_facmActvLane) -> Divide2/2  "MPInP_phiPrvwHdAgIni"
  Divide2/1 -> Add/2
  Lane Information Selection (LaneInfoSel)1/1(LaneInfoSel_facmActvLane) -> Add/1  "MPInP_lDvtIni"
  Lane Information Selection (LaneInfoSel)2/1(LaneInfoSel_facmActvLane) -> Signal Latching3/1(In)  "MPInP_lDvtIni"
  Bus Selector4/4 -> Gain/1  "<UndrLim_dphiSWARMax>"
  Bus Selector4/10 -> Lane Information Selection (LaneInfoSel)2/3(LaneInfoSel_facmRgtLane)  "<lPrvwDvtRgt>"
  Bus Selector4/9 -> Lane Information Selection (LaneInfoSel)2/2(LaneInfoSel_facmLftLane)  "<lPrvwDvtLft>"
  Bus Selector4/8 -> Lane Information Selection (LaneInfoSel)1/5(LaneInfoSel_phiPrvwTTLCHdAgRgtTTLCRgt)  "<phiPrvwTTLCHdAgRgtTTLCRgt>"
  Bus Selector4/5 -> Lane Information Selection (LaneInfoSel)1/2(LaneInfoSel_phiPrvwTTLCHdAgLftTTLCLft)  "<phiPrvwTTLCHdAgLftTTLCLft>"
  Saturation3/1 -> Divide1/2  "Vx"
  Constant/1 -> Divide1/1
  Saturation2/1 -> Bus Creator/2  "MPInP_tiTTLCIni"
  Bus Creator/1 -> MPInP_bsMPInPInfo/1
  Divide1/1 -> Saturation1/1
  Subsystem/1(Out6) -> Bus Creator/1  "MPInP_stLDDir"
  MPInP_bsInInfoSyn/1 -> Bus Selector3/1
  Bus Selector3/2 -> Signal Latching7/1(In), Cast To Single1/1, Saturation3/1  "<ESC_VehSpd>"
  Signal Latching7/1(Out) -> Bus Creator/9  "MPInP_vVehSpdIni"
  Signal Latching5/1(Out) -> Saturation2/1  "MPInP_tiTTLCIni"
  Saturation1/1 -> Bus Creator/11  "MPInP_StbFacm_SY"
  MPInP_stLKAActvFlg/1 -> Subsystem/1(In1), Lane Information Selection (LaneInfoSel)/1(LaneInfoSel_stLKAActvFlg), Lane Information Selection (LaneInfoSel)3/1(LaneInfoSel_stLKAActvFlg), Lane Information Selection (LaneInfoSel)1/1(LaneInfoSel_stLKAActvFlg), Lane Information Selection (LaneInfoSel)4/1(LaneInfoSel_stLKAActvFlg), Lane Information Selection (LaneInfoSel)2/1(LaneInfoSel_stLKAActvFlg)
  Signal Latching3/1(Out) -> Bus Creator/4  "MPInP_lDvtIni"
  Signal Latching2/1(Out) -> Bus Creator/3  "MPInP_phiPrvwHdAgIni"
  Signal Latching4/1(Out) -> Bus Creator/5  "MPInP_phiHdAgIni"
  MPInP_phiHdAgMax/1 -> Signal Latching/1(In)  "MPInP_phiHdAgMax"
  Bus Selector3/1 -> Add1/1  "<SW_Angle>"
  Cast To Single1/1 -> Bus Creator/10  "MPInP_vVehSpd"
  MPInP_bsLKAInPInfo/1 -> Bus Selector1/1, Bus Selector4/1
  Lane Information Selection (LaneInfoSel)/1(LaneInfoSel_facmActvLane) -> Signal Latching5/1(In)
  Bus Selector1/1 -> Lane Information Selection (LaneInfoSel)/2(LaneInfoSel_facmLftLane)  "<LFTTTLC>"
  Bus Selector1/2 -> Lane Information Selection (LaneInfoSel)/3(LaneInfoSel_facmRgtLane)  "<RGTTTLC>"
  Signal Latching6/1(Out) -> Bus Creator/8  "MPInP_phiSWAIni"
  Signal Latching/1(Out) -> Bus Creator/7  "MPInP_phiHdAgMax"

== system LKAS_AutoSave_DF_20220408_1006_SW62/LKAS/LL/LLOn/LKA/LKA Motion Planning (LKAMP) /Nominal Time Calculation (NomTCalc) ==
  NomTCalc_vVehSpd : Inport
  NomTCalc_vVehSpdIni : Inport  Port=2
  Add : Sum  OutDataTypeStr=single
  Divide : Product  Inputs=*/  OutDataTypeStr=single
  Gain : Gain  Gain=1/3.6  OutDataTypeStr=single
  Gain1 : Gain  Gain=1/3.6  OutDataTypeStr=single
  Memory : Memory  InheritSampleTime=on
  Product : Product
  NomTCalc_tiNomT : Outport
  wires:
  NomTCalc_vVehSpd/1 -> Gain/1
  Add/1 -> NomTCalc_tiNomT/1, Memory/1
  Memory/1 -> Add/2
  Gain/1 -> Product/1
  NomTCalc_vVehSpdIni/1 -> Gain1/1
  Gain1/1 -> Divide/2
  Product/1 -> Divide/1
  Divide/1 -> Add/1
  [LKA_SampleTime] -> Product/2

== system LKAS_AutoSave_DF_20220408_1006_SW62/LKAS/LL/LLOn/LKA/LKA Motion Planning (LKAMP) /Steering Wheel Angle Command Calculation (SWACmdCal) ==
  SWACmdCal_bsK1K2DetOut : Inport
  SWACmdCal_bsLKAInPInfo : Inport  Port=2
  SWACmdCal_tiNomT : Inport  Port=3
  Bus Selector : BusSelector  OutputSignals=K1K2Det_dphi1PhSWAGrad,K1K2Det_phi2PhSWAIni,K1K2Det_T1
  Bus Selector1 : BusSelector  OutputSignals=MPInP_phiSWAIni
  SWACmd : MATLAB Function  TreatAsAtomicUnit=on
  SWACmd1 : MATLAB Function  Commented=on  TreatAsAtomicUnit=on
  SWACmdCal_phiSWACmd : Outport
  SWACmdCal_tiT1 : Outport  Port=2
  wires:
  Bus Selector/3 -> SWACmd/3(K1K2Det_T1)  "<K1K2Det_T1>"
  SWACmd/2(T1) -> SWACmdCal_tiT1/1
  SWACmdCal_tiNomT/1 -> SWACmd/5(SWACmd_tiNomT)
  Bus Selector1/1 -> SWACmd/4(SWACmd_phi1PhSWAIni)  "<MPInP_phiSWAIni>"
  SWACmdCal_bsLKAInPInfo/1 -> Bus Selector1/1
  Bus Selector/1 -> SWACmd/1(SWACmd_dphi1PhSWAGrad)  "<K1K2Det_dphi1PhSWAGrad>"
  Bus Selector/2 -> SWACmd/2(SWACmd_phi2PhSWAIni)  "<K1K2Det_phi2PhSWAIni>"
  SWACmdCal_bsK1K2DetOut/1 -> Bus Selector/1
  SWACmd/1(SWACmd_phiSWACmd) -> SWACmdCal_phiSWACmd/1

== system LKAS_AutoSave_DF_20220408_1006_SW62/LKAS/LL/LLOn/LKA/LKA Motion Planning (LKAMP) /Switching Condition (SwtCon) ==
  SwtCon_stLKAActvFlg : Inport
  SwtCon_bsLKAInPInfo : Inport  Port=2
  SwtCon_vVehSpd : Inport  Port=3
  SwtCon_lLaneWidth_C : Inport  Port=4
  SwtCon_lCarWidth_C : Inport  Port=5
  SwtCon_tiHdAgExTime_C : Inport  Port=6
  SwtCon_tiLSpdCompT_C : Inport  Port=7
  Bus Selector1 : BusSelector  OutputSignals=bsPrCrvtInfo.crPrvwCrvt
  Ending Heading Angle Determination (EndHdAgDet) : Subsystem
  If : If  IfExpression=u1==1  ElseIfExpressions=u1==2
  If Action Subsystem : Subsystem  TreatAsAtomicUnit=on
  If Action Subsystem1 : Subsystem  TreatAsAtomicUnit=on
  If Action Subsystem2 : Subsystem  TreatAsAtomicUnit=on
  Merge : Merge  Inputs=3
  SwtCon_phiHdAgMax : Outport
  wires:
  If/1 -> If Action Subsystem/Action
  If Action Subsystem/1(Out1) -> Merge/1
  If/2 -> If Action Subsystem1/Action
  If Action Subsystem1/1(Out1) -> Merge/2
  If/3 -> If Action Subsystem2/Action
  If Action Subsystem2/1(Out1) -> Merge/3
  SwtCon_lLaneWidth_C/1 -> Ending Heading Angle Determination (EndHdAgDet)/4(EndHdAgDet_lLaneWidth_C)
  SwtCon_lCarWidth_C/1 -> Ending Heading Angle Determination (EndHdAgDet)/5(EndHdAgDet_lCarWidth_C)
  SwtCon_tiHdAgExTime_C/1 -> Ending Heading Angle Determination (EndHdAgDet)/6(EndHdAgDet_tiHdAgExTime_C)
  SwtCon_vVehSpd/1 -> Ending Heading Angle Determination (EndHdAgDet)/2(EndHdAgDet_vVehSpd)
  Ending Heading Angle Determination (EndHdAgDet)/1(EndHdAgDet_phiHdAgMax) -> If Action Subsystem1/1(In1), If Action Subsystem/1(In1)
  SwtCon_stLKAActvFlg/1 -> If/1, Ending Heading Angle Determination (EndHdAgDet)/1(EndHdAgDet_stLKAActvFlg)
  Merge/1 -> SwtCon_phiHdAgMax/1
  SwtCon_tiLSpdCompT_C/1 -> Ending Heading Angle Determination (EndHdAgDet)/7(EndHdAgDet_tiLSpdCompT_C)
  SwtCon_bsLKAInPInfo/1 -> Bus Selector1/1
  Bus Selector1/1 -> Ending Heading Angle Determination (EndHdAgDet)/3(EndHdAgDet_crPrvwCrvt)  "<crPrvwCrvt>"

== system LKAS_AutoSave_DF_20220408_1006_SW62/LKAS/LL/LLOn/LKA/LKA Motion Planning (LKAMP) /Trigger Once ==
  Add : Sum  OutDataTypeStr=uint8
  Constant : Constant  OutDataTypeStr=uint8  SampleTime=-1
  Constant19 : Constant  OutDataTypeStr=uint8  SampleTime=-1
  If : If  NumInputs=2  IfExpression=u1==u2  ShowElse=off
  Memory1 : Memory  InheritSampleTime=on
  Saturation1 : Saturate  UpperLimit=5  LowerLimit=0  OutDataTypeStr=uint8
      settings: AttributesFormatString="Min = %<LowerLimit>  Max = %<UpperLimit>"
  Out1 : Outport
  wires:
  Constant19/1 -> If/2
  Add/1 -> Saturation1/1
  If/1 -> Out1/1
  Memory1/1 -> Add/2
  Saturation1/1 -> If/1, Memory1/1
  Constant/1 -> Add/1

== system LKAS_AutoSave_DF_20220408_1006_SW62/LKAS/LL/LLOn/LKA/LKA SWA Limit (LKASWALim)/Rate Limiter Dynamic  ==
  note: U(k)
  note: Y(k)
  up : Inport
  u : Inport  Port=2
  lo : Inport  Port=3
  Add1 : Sum  OutDataTypeStr=uint16
  Constant : Constant  OutDataTypeStr=uint16  SampleTime=-1
  Delay Input2 : UnitDelay  Description=Store in Global RAM  DisableCoverage=on  SampleTime=-1
  Difference Inputs1 : Sum  Description=Add in CPU  DisableCoverage=on  Inputs=+-  OutDataTypeStr=Inherit: Inherit via back propagation
  Difference Inputs2 : Sum  Description=Add in CPU  OutDataTypeStr=Inherit: Inherit via back propagation
  LatchTime_SY : Constant  OutDataTypeStr=uint16  SampleTime=-1
  Memory : Memory  InheritSampleTime=on
  Relational Operator : RelationalOperator  Operator=<=  OutDataTypeStr=boolean  RndMeth=Nearest
  Saturation Dynamic : simulink/Discontinuities/Saturation Dynamic  OutMin=[]  OutMax=[]  OutDataTypeStr=Inherit: Same as second input  OutDataType=fixdt(1, 16)  OutScaling=2^-10  DoSatur=off
  Saturation2 : Saturate  UpperLimit=10000  LowerLimit=0  OutDataTypeStr=uint16
      settings: AttributesFormatString="Min = %<LowerLimit>  Max = %<UpperLimit>"
  Switch : Switch  Criteria=u2 > Threshold
  delta fall limit : Product  DisableCoverage=on  Inputs=**  OutDataTypeStr=Inherit: Inherit via back propagation  SaturateOnIntegerOverflow=on
  delta rise limit : Product  DisableCoverage=on  Inputs=**  OutDataTypeStr=Inherit: Inherit via back propagation  SaturateOnIntegerOverflow=on
  sample time : SampleTimeMath  DisableCoverage=on  TsampMathOp=Ts Only  weightValue=1
  Y : Outport
  wires:
  Delay Input2/1 -> Switch/3  "Y(k-1)"
  Relational Operator/1 -> Switch/2
  Constant/1 -> Add1/1
  LatchTime_SY/1 -> Relational Operator/2
  Saturation2/1 -> Memory/1
  Memory/1 -> Add1/2
  Add1/1 -> Saturation2/1, Relational Operator/1
  delta fall limit/1 -> Saturation Dynamic/3
  Difference Inputs1/1 -> Saturation Dynamic/2  "( U(k) - Y(k-1) )"
  Switch/1 -> Difference Inputs1/2, Difference Inputs2/2  "Y(k-1)"
  Saturation Dynamic/1 -> Difference Inputs2/1
  Difference Inputs2/1 -> Delay Input2/1, Y/1
  delta rise limit/1 -> Saturation Dynamic/1
  up/1 -> delta rise limit/1
  lo/1 -> delta fall limit/1
  sample time/1 -> delta rise limit/2, delta fall limit/2
  u/1 -> Difference Inputs1/1, Switch/1, sample time/1

== system LKAS_AutoSave_DF_20220408_1006_SW62/LKAS/LL/LLOn/LKA/Lane Following (LF)/Preview Information Calculation (PIC) ==
  PIC_bsLKAInPInfo : Inport
  Bus Creator : BusCreator  Inputs=6
  Bus Selector1 : BusSelector  OutputSignals=bsPrDvtInfo.lPrvwDvtMean,bsPrHdAgInfo.phiPrvwHdAgMean,bsPrCrvtInfo.crPrvwCrvtMean,LaneWidth,bsPrHdAgInfo.PrvwZMean,bsPrCrvtInfo.crPrvwCrvtMean
  PIC_bsPrvwInfo : Outport
  wires:
  Bus Selector1/6 -> Bus Creator/6  "<crPrvwCrvtMean>"
  Bus Selector1/5 -> Bus Creator/5  "<PrvwZMean>"
  Bus Selector1/1 -> Bus Creator/1  "<lPrvwDvtMean>"
  Bus Selector1/2 -> Bus Creator/2  "<phiPrvwHdAgMean>"
  Bus Selector1/3 -> Bus Creator/3  "<crPrvwCrvtMean>"
  PIC_bsLKAInPInfo/1 -> Bus Selector1/1
  Bus Creator/1 -> PIC_bsPrvwInfo/1
  Bus Selector1/4 -> Bus Creator/4  "<LaneWidth>"
